simulink model "ChevNAOveleves"  (R2015b)
settings: Solver=ode45  StartTime=0.0  StopTime=1  MaxStep=0.01  RelTol=1e-3
values from neighbouring files (symbols this model uses):
  Cext = 0    [ParamChev.m]
  Ki = 0.0194    [ParamChev.m]
undefined symbols (not defined in the file or in its folder): Kd, Kp
settings Model: Creator=antomart  LastModifiedBy=David
settings DataIOCC: LimitDataPoints=off  SaveFormat=StructureWithTime
settings HardwareCC: ProdWordSize=32  ProdHWDeviceType=Specified
settings ModelReferenceCC: PropagateSignalLabelsOutOfModel=on
settings GRTTargetCC: GeneratePreprocessorConditionals=Disable all

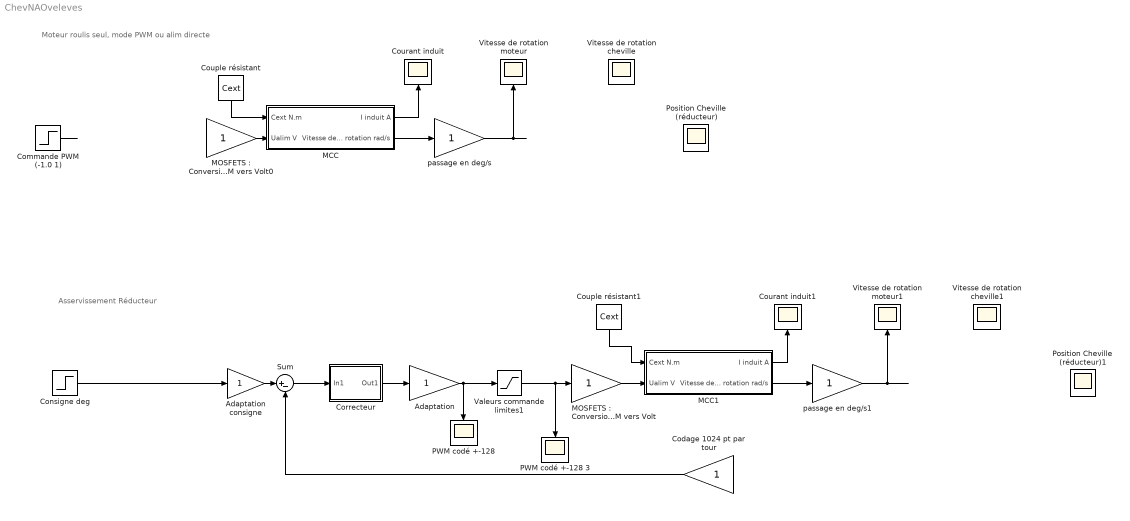
== system ChevNAOveleves ==
  note: Asservissement Réducteur
  note: Moteur roulis seul, mode PWM ou alim directe
  Adaptation : Gain
  Adaptation consigne : Gain
  Codage 1024 pt par tour : Gain
  Commande PWM (-1.0 1) : Step  Time=0  After=0.5  SampleTime=0
  Consigne deg : Step  Time=0  After=30  SampleTime=0
  Correcteur : Subsystem
  Couple résistant : Constant  Value=Cext
  Couple résistant1 : Constant  Value=Cext
  Courant induit : Scope
  Courant induit1 : Scope
  MCC : Subsystem
  MCC1 : Subsystem
  "MOSFETS : Conversion PWM vers Volt" : Gain
  "MOSFETS : Conversion PWM vers Volt0" : Gain
  PWM codé +-128 3 : Scope
  PWM codé +-128 : Scope
  Position Cheville (réducteur) : Scope
  Position Cheville (réducteur)1 : Scope
  Sum : Sum  Inputs=|+-
  Valeurs commande limites1 : Saturate  UpperLimit=1  LowerLimit=1
  Vitesse de rotation cheville : Scope
  Vitesse de rotation cheville1 : Scope
  Vitesse de rotation moteur : Scope
  Vitesse de rotation moteur1 : Scope
  passage en deg/s : Gain
  passage en deg/s1 : Gain
  wires:
  Couple résistant/1 -> MCC/1(Cext N.m)
  MCC/1(I induit A) -> Courant induit/1
  MCC/2(Vitesse de rotation rad/s) -> passage en deg/s/1
  passage en deg/s/1 -> Vitesse de rotation moteur/1
  ? -> Vitesse de rotation cheville/1
  Couple résistant1/1 -> MCC1/1(Cext N.m)
  MCC1/1(I induit A) -> Courant induit1/1
  MCC1/2(Vitesse de rotation rad/s) -> passage en deg/s1/1
  passage en deg/s1/1 -> Vitesse de rotation moteur1/1
  ? -> Position Cheville (réducteur)/1
  ? -> Vitesse de rotation cheville1/1
  ? -> Codage 1024 pt par tour/1, Position Cheville (réducteur)1/1
  "MOSFETS : Conversion PWM vers Volt0"/1 -> MCC/2(Ualim V)
  ? -> "MOSFETS : Conversion PWM vers Volt0"/1
  Valeurs commande limites1/1 -> PWM codé +-128 3/1, "MOSFETS : Conversion PWM vers Volt"/1
  "MOSFETS : Conversion PWM vers Volt"/1 -> MCC1/2(Ualim V)
  Sum/1 -> Correcteur/1(In1)
  Correcteur/1(Out1) -> Adaptation/1
  Adaptation/1 -> Valeurs commande limites1/1, PWM codé +-128/1
  Consigne deg/1 -> Adaptation consigne/1
  Commande PWM (-1.0 1)/1 -> ?
  Codage 1024 pt par tour/1 -> Sum/2
  Adaptation consigne/1 -> Sum/1

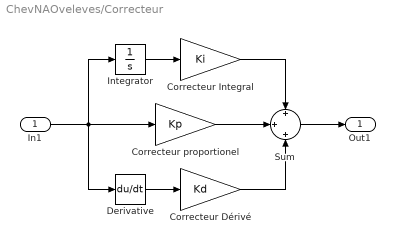
== system ChevNAOveleves/Correcteur ==
  In1 : Inport
  Correcteur Dérivé : Gain  Gain=Kd
  Correcteur Integral : Gain  Gain=Ki
  Correcteur proportionel : Gain  Gain=Kp
  Derivative : Derivative
  Integrator : Integrator
  Sum : Sum  Inputs=+|+|+
  Out1 : Outport
  wires:
  In1/1 -> Derivative/1, Integrator/1, Correcteur proportionel/1
  Integrator/1 -> Correcteur Integral/1
  Correcteur Integral/1 -> Sum/1
  Correcteur proportionel/1 -> Sum/2
  Derivative/1 -> Correcteur Dérivé/1
  Correcteur Dérivé/1 -> Sum/3
  Sum/1 -> Out1/1

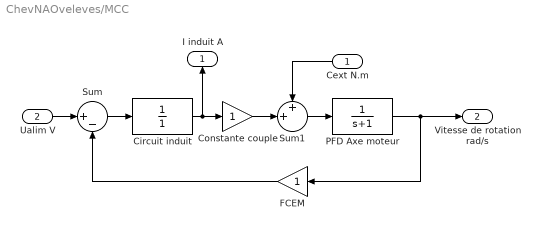
== system ChevNAOveleves/MCC ==
  Cext N.m : Inport
  Ualim V : Inport  Port=2
  Circuit induit : TransferFcn  Denominator=[0 1]
  Constante couple : Gain
  FCEM : Gain
  PFD Axe moteur : TransferFcn  Denominator=[1 1]
  Sum : Sum  Inputs=|+-
  Sum1 : Sum  Inputs=++|
  I induit A : Outport
  Vitesse de rotation rad/s : Outport  Port=2
  wires:
  PFD Axe moteur/1 -> Vitesse de rotation rad/s/1, FCEM/1
  Sum1/1 -> PFD Axe moteur/1
  Constante couple/1 -> Sum1/2
  Circuit induit/1 -> Constante couple/1, I induit A/1
  Sum/1 -> Circuit induit/1
  FCEM/1 -> Sum/2
  Cext N.m/1 -> Sum1/1
  Ualim V/1 -> Sum/1

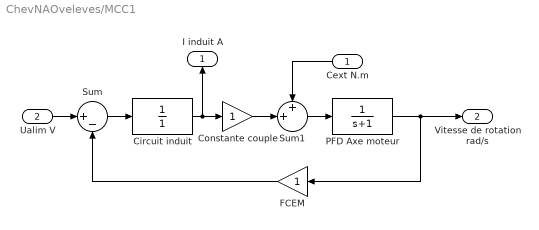
== system ChevNAOveleves/MCC1 ==
  Cext N.m : Inport
  Ualim V : Inport  Port=2
  Circuit induit : TransferFcn  Denominator=[0 1]
  Constante couple : Gain
  FCEM : Gain
  PFD Axe moteur : TransferFcn  Denominator=[1 1]
  Sum : Sum  Inputs=|+-
  Sum1 : Sum  Inputs=++|
  I induit A : Outport
  Vitesse de rotation rad/s : Outport  Port=2
  wires:
  PFD Axe moteur/1 -> Vitesse de rotation rad/s/1, FCEM/1
  Sum1/1 -> PFD Axe moteur/1
  Constante couple/1 -> Sum1/2
  Circuit induit/1 -> Constante couple/1, I induit A/1
  Sum/1 -> Circuit induit/1
  FCEM/1 -> Sum/2
  Cext N.m/1 -> Sum1/1
  Ualim V/1 -> Sum/1
